simulink model "rtwdemo_advisor2"  (Simulink 7.6)
settings: Solver=FixedStepDiscrete  SolverMode=SingleTasking  StartTime=0.0  StopTime=4  FixedStep=1  RelTol=1e-3  AbsTol=1e-6
libraries: simulink_need_slupdate x2, rtwdemowidgets x1
Description:
  | Using Model Advisor for optimizing the model for real-time deployment
settings Model: Creator=The MathWorks Inc.  CovMetricSettings=d  ExtModeTrigMode=oneshot  ExtModeArmWhenConnect=off  ExtModeAutoUpdateStatusClock=off
settings MATStruct: SampleTime=1  Offset=0  Priority=[20.0]
settings DataIOCC: LimitDataPoints=off  SaveOutput=off  SaveTime=off  SignalLoggingName=sigsOut
settings OptimizationCC: InlineParams=on  InlineInvariantSignals=on  PassReuseOutputArgsAs=Individual arguments  StateBitsets=on  DataBitsets=on  UseTempVars=on  ZeroExternalMemoryAtStartup=off  ZeroInternalMemoryAtStartup=off  NoFixptDivByZeroProtection=on  EfficientFloat2IntCast=on  EfficientMapNaN2IntZero=off  OptimizeModelRefInitCode=on  LifeSpan=1  BufferReusableBoundary=off
settings DebuggingCC: CheckExecutionContextPreStartOutputMsg=on  CheckExecutionContextRuntimeOutputMsg=on  SolverPrmCheckMsg=none  IntegerOverflowMsg=none  ParameterDowncastMsg=warning  ParameterOverflowMsg=warning  ParameterPrecisionLossMsg=none  StrictBusMsg=ErrorOnBusTreatedAsVector
settings HardwareCC: ProdIntDivRoundTo=Zero  ProdEndianess=LittleEndian  ProdHWDeviceType=Generic->32-bit Embedded Processor  TargetHWDeviceType=Generic->32-bit Embedded Processor
settings SFSimCC: SimParseCustomCode=off
settings RTWCC: SystemTargetFile=ert.tlc  GenCodeOnly=on  TemplateMakefile=ert_default_tmf  GenerateReport=on  RTWVerbose=off  ProcessScript=ert_make_rtw_hook  IncludeHyperlinkInReport=on  LaunchReport=on
settings CodeAppCC: IgnoreCustomStorageClasses=off  IgnoreTestpoints=on  IncHierarchyInIds=on  IncDataTypeInIds=on  InlinedPrmAccess=Macros
settings ERTTargetCC: TargetFcnLib=ansi_tfl_tmw.mat  MultiwordLength=2048  GenerateSampleERTMain=on  SupportNonFinite=off  ERTCustomFileTemplate=example_file_process.tlc  ConvertIfToSwitch=off

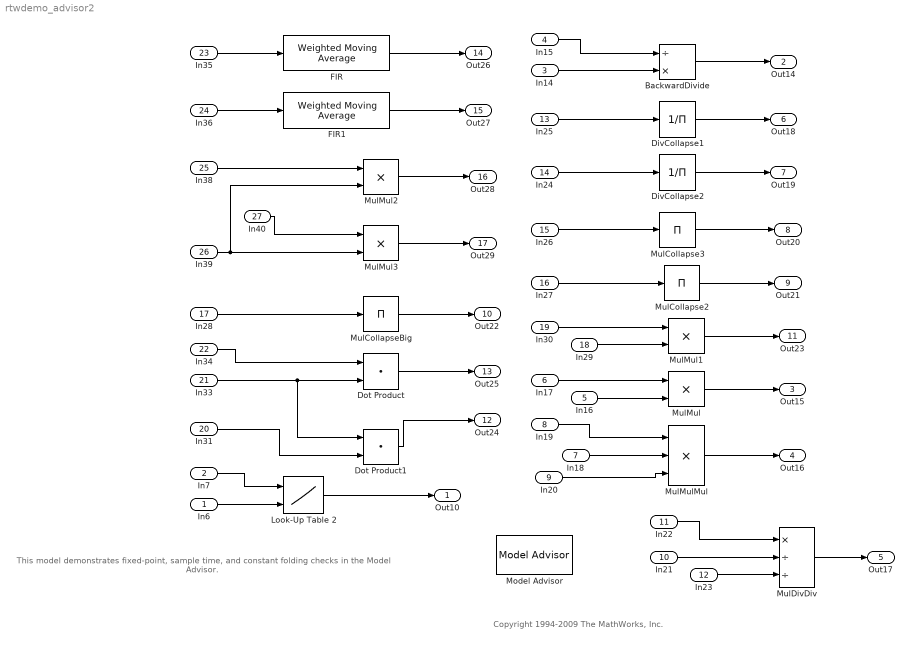
== system rtwdemo_advisor2 ==
  note: This model demonstrates fixed-point,
      | sample time, and constant folding checks
      | in the Model Advisor.
  note: Copyright 1994-2009 The MathWorks, Inc.
  In6 : Inport  OutDataTypeStr=fixdt(1,16,10)  PortDimensions=1  SampleTime=1  Interpolate=off
  In7 : Inport  Port=2  OutDataTypeStr=fixdt(1,16,10)  PortDimensions=1  SampleTime=1  Interpolate=off
  In14 : Inport  Port=3  OutDataTypeStr=fixdt(1,16,10)  PortDimensions=1  SampleTime=1  Interpolate=off
  In15 : Inport  Port=4  OutDataTypeStr=fixdt(1,16,10)  PortDimensions=1  SampleTime=1  Interpolate=off
  In16 : Inport  Port=5  OutDataTypeStr=fixdt(1,32,10)  PortDimensions=1  SampleTime=1  Interpolate=off
  In17 : Inport  Port=6  OutDataTypeStr=fixdt(1,16,10)  PortDimensions=1  SampleTime=1  Interpolate=off
  In18 : Inport  Port=7  OutDataTypeStr=fixdt(1,16,10)  PortDimensions=1  SampleTime=1  Interpolate=off
  In19 : Inport  Port=8  OutDataTypeStr=fixdt(1,16,10)  PortDimensions=1  SampleTime=1  Interpolate=off
  In20 : Inport  Port=9  OutDataTypeStr=fixdt(1,16,10)  PortDimensions=1  SampleTime=1  Interpolate=off
  In21 : Inport  Port=10  OutDataTypeStr=fixdt(1,16,10)  PortDimensions=1  SampleTime=1  Interpolate=off
  In22 : Inport  Port=11  OutDataTypeStr=fixdt(1,16,10)  PortDimensions=1  SampleTime=1  Interpolate=off
  In23 : Inport  Port=12  OutDataTypeStr=fixdt(1,16,10)  PortDimensions=1  SampleTime=1  Interpolate=off
  In25 : Inport  Port=13  OutDataTypeStr=fixdt(1,16,10)  PortDimensions=1  SampleTime=1  Interpolate=off
  In24 : Inport  Port=14  OutDataTypeStr=fixdt(1,16,10)  PortDimensions=2  SampleTime=1  Interpolate=off
  In26 : Inport  Port=15  OutDataTypeStr=fixdt(1,16,10)  PortDimensions=3  SampleTime=1  Interpolate=off
  In27 : Inport  Port=16  OutDataTypeStr=fixdt(1,16,10)  PortDimensions=2  SampleTime=1  Interpolate=off
  In28 : Inport  Port=17  OutDataTypeStr=fixdt(1,32,10)  PortDimensions=2  SampleTime=1  Interpolate=off
  In29 : Inport  Port=18  OutDataTypeStr=fixdt(1,16,10)  PortDimensions=1  SampleTime=1  Interpolate=off
  In30 : Inport  Port=19  OutDataTypeStr=fixdt(1,16,10)  PortDimensions=1  SampleTime=1  Interpolate=off
  In31 : Inport  Port=20  OutDataTypeStr=fixdt(1,32,10)  PortDimensions=1  SampleTime=1  Interpolate=off
  In33 : Inport  Port=21  OutDataTypeStr=fixdt(1,16,10)  PortDimensions=1  SampleTime=1  Interpolate=off
  In34 : Inport  Port=22  OutDataTypeStr=fixdt(1,16,10)  PortDimensions=1  SampleTime=1  Interpolate=off
  In35 : Inport  Port=23  OutDataTypeStr=fixdt(1,32,10)  PortDimensions=1  SampleTime=1  Interpolate=off
  In36 : Inport  Port=24  OutDataTypeStr=fixdt(1,32,10)  PortDimensions=1  SampleTime=1  Interpolate=off
  In38 : Inport  Port=25  OutDataTypeStr=fixdt(1, 16, 1.01 * 2^-10, 0)  PortDimensions=1  SampleTime=1  Interpolate=off
  In39 : Inport  Port=26  OutDataTypeStr=fixdt(1,16,10)  PortDimensions=1  SampleTime=1  Interpolate=off
  In40 : Inport  Port=27  OutDataTypeStr=fixdt(1, 16, 2^-10,1)  PortDimensions=1  SampleTime=1  Interpolate=off
  BackwardDivide : Product  Inputs=/*  OutDataTypeStr=fixdt(1,16,10)
  DivCollapse1 : Product  Inputs=/  OutDataTypeStr=fixdt(1,16,10)
  DivCollapse2 : Product  Inputs=/  OutDataTypeStr=fixdt(1,16,10)
  Dot Product : DotProduct  OutDataTypeStr=fixdt(1,32,10)
  Dot Product1 : DotProduct  OutDataTypeStr=fixdt(1,32,10)
  FIR : simulink_need_slupdate/Weighted Moving Average  mgainval=[0.1:0.1:1 0.9:-0.1:0.1]  vinit=0.0  samptime=-1  OutDataTypeStr=fixdt(1,32,10)  OutputDataTypeScalingMode=Specify via dialog  OutDataType=sfix(32)  OutScaling=2^-10  DoSatur=off  GainDataTypeStr=sfix( 16 )  GainDataTypeScalingMode=Specify via dialog  GainDataType=sfix( 16 )  MatRadixGroup=Best Precision: Matrix-wise  GainScaling=2^-14
  FIR1 : simulink_need_slupdate/Weighted Moving Average  mgainval=[0.1:0.1:1 0.9:-0.1:0.1]  vinit=0.0  samptime=-1  OutDataTypeStr=fixdt(1,32,20)  OutputDataTypeScalingMode=Specify via dialog  OutDataType=sfix(32)  OutScaling=2^-20  DoSatur=off  GainDataTypeStr=sfix( 16 )  GainDataTypeScalingMode=Specify via dialog  GainDataType=sfix( 16 )  MatRadixGroup=Best Precision: Matrix-wise  GainScaling=2^-14
  Look-Up Table 2 : Lookup2D  RowIndex=[1:3]  ColumnIndex=[1 2 7]  Table=[4 5 6;16 19 20;10 18 23]  LookUpMeth=Interpolation-Use End Values  OutDataTypeStr=fixdt(1,16,10)
  Model Advisor : rtwdemowidgets/Model Advisor  SystemSampleTime=-1  attrib_overrides={}
  MulCollapse2 : Product  Inputs=1  OutDataTypeStr=fixdt(1,16,10)
  MulCollapse3 : Product  Inputs=*  OutDataTypeStr=fixdt(1,16,10)
  MulCollapseBig : Product  Inputs=1  OutDataTypeStr=fixdt(1,16,10)
  MulDivDiv : Product  Inputs=*//  OutDataTypeStr=fixdt(1,16,10)
  MulMul : Product  OutDataTypeStr=fixdt(1,16,3)
  MulMul1 : Product  OutDataTypeStr=fixdt(1,16,10)
  MulMul2 : Product  OutDataTypeStr=fixdt(1,16,10)
  MulMul3 : Product  OutDataTypeStr=fixdt(1,16,10)
  MulMulMul : Product  Inputs=3  OutDataTypeStr=fixdt(1,16,10)
  Out10 : Outport
  Out14 : Outport  Port=2
  Out15 : Outport  Port=3
  Out16 : Outport  Port=4
  Out17 : Outport  Port=5
  Out18 : Outport  Port=6
  Out19 : Outport  Port=7
  Out20 : Outport  Port=8
  Out21 : Outport  Port=9
  Out22 : Outport  Port=10
  Out23 : Outport  Port=11
  Out24 : Outport  Port=12
  Out25 : Outport  Port=13
  Out26 : Outport  Port=14
  Out27 : Outport  Port=15
  Out28 : Outport  Port=16
  Out29 : Outport  Port=17
  wires:
  In6/1 -> Look-Up Table 2/2
  Look-Up Table 2/1 -> Out10/1
  In7/1 -> Look-Up Table 2/1
  In14/1 -> BackwardDivide/2
  BackwardDivide/1 -> Out14/1
  In15/1 -> BackwardDivide/1
  MulMul/1 -> Out15/1
  In17/1 -> MulMul/1
  In18/1 -> MulMulMul/2
  MulMulMul/1 -> Out16/1
  In19/1 -> MulMulMul/1
  In20/1 -> MulMulMul/3
  In21/1 -> MulDivDiv/2
  MulDivDiv/1 -> Out17/1
  In22/1 -> MulDivDiv/1
  In23/1 -> MulDivDiv/3
  DivCollapse1/1 -> Out18/1
  In25/1 -> DivCollapse1/1
  DivCollapse2/1 -> Out19/1
  In24/1 -> DivCollapse2/1
  MulCollapse3/1 -> Out20/1
  In26/1 -> MulCollapse3/1
  MulCollapse2/1 -> Out21/1
  In27/1 -> MulCollapse2/1
  MulCollapseBig/1 -> Out22/1
  In28/1 -> MulCollapseBig/1
  MulMul1/1 -> Out23/1
  In30/1 -> MulMul1/1
  In31/1 -> Dot Product1/2
  Dot Product1/1 -> Out24/1
  In33/1 -> Dot Product/2, Dot Product1/1
  Dot Product/1 -> Out25/1
  In34/1 -> Dot Product/1
  In35/1 -> FIR/1
  FIR/1 -> Out26/1
  In36/1 -> FIR1/1
  FIR1/1 -> Out27/1
  MulMul2/1 -> Out28/1
  In38/1 -> MulMul2/1
  In39/1 -> MulMul3/2, MulMul2/2
  MulMul3/1 -> Out29/1
  In40/1 -> MulMul3/1
  In16/1 -> MulMul/2
  In29/1 -> MulMul1/2
